simulink library "forceslib"  (R2019b)
settings: Solver=VariableStepAuto  StartTime=0.0  StopTime=10.0  RelTol=1e-3
undefined symbols (not defined in the file or in its folder): MV0, X0
settings Model: Creator=rchen  LastModifiedBy=j-hho

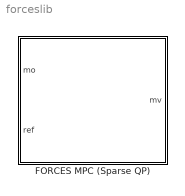
== system forceslib ==
  FORCES MPC (Sparse QP) : Subsystem  InitFcn=forcesmpcblock_InitFcn  mask(ForcesMPC_SparseQP){CoreData=[], StateData=[], md_inport=off, mv_inport=off, uref_inport=off, state_inport=off, ymin_inport=off, ymax_inport=off, umin_inport=off, umax_inport=off, dumin_inport=off, dumax_inport=off, ywt_inport=off, uwt_inport=off, duwt_inport=off, ecrwt_inport=off, return_cost=off, return_mvseq=off, return_qpstatus=off, return_xseq=off, return_state=off, return_yseq=off}
      mask prompts: CoreData "Core Data"; StateData "Initial State Data"; md_inport "Measured disturbance (md)"; mv_inport "External manipulated variable (ext.mv)"; uref_inport "References for manipulated variables (mv.target)"; state_inport "Use custom state estimation (x[k|k])"; ymin_inport "Lower OV Limits (ymin)"; ymax_inport "Upper OV Limits (ymax)"; umin_inport "Lower MV Limits (umin)"; umax_inport "Upper MV Limits (umax)"; dumin_inport "Lower MVRate Limits (dumin)"; dumax_inport "Upper MVRate Limits (dumax)"; ywt_inport "OV Weights (y.wt)"; uwt_inport "MV Weights (u.wt)"; duwt_inport "MVRate Weights (du.wt)"; ecrwt_inport "Slack Variable Weight (ecr.wt)"; return_cost "Optimal cost (cost)"; return_mvseq "Optimal control sequence (mv.seq)"; return_qpstatus "Optimization status (qp.status)"; return_xseq "Optimal state sequence (x.seq)"; return_state "Estimated current states (est.state)"; return_yseq "Optimal output sequence (y.seq)"
      mask help:
      | Simulate MPC controller and generate code  using FORCES QP solver.
      |
      | In MATLAB, use the following commands to generate custom FORCES QP solver from your MPC controller (mpcobj):
      |     options = mpcToForcesOptions('sparse');
      |     [coredata, statedata, onlinedata] = mpcToForces(mpcobj, options);
      | You can enable additional online features via the "options".
      |
      | Afterwards, specify "coredata" and "statedata" in the block dialog and enable additional input and output signals in the block that must be consistent with "options".
      mask init:
      | [blk, Ts, MPCstruct, X0, MV0] = forcesmpcblock_MaskInitFcnParameter;
      | if isempty(MPCstruct)
      |     forcesmpcblock_MaskInitFcnResize(blk,0,1,1,1);
      | else
      |     forcesmpcblock_MaskInitFcnResize(blk,MPCstruct.nmd,MPCstruct.nmv,MPCstruct.ny,MPCstruct.nmy);
      | end
      mask DialogControl Container5 Prompt: Additional Signal Configuration
      mask DialogControl Container7 Prompt: State Estimation
      mask DialogControl Container3 Prompt: Online Constraints
      mask DialogControl Container4 Prompt: Online Weights
      mask DialogControl Container9 Prompt: Additional Output Signals
      mask Display:
      | fprintf('FORCES MPC\n\n(Sparse QP)');
      | port_label('output', 1, 'mv')
      | port_label('input', 1, 'mo')
      | port_label('input', 2, 'ref')

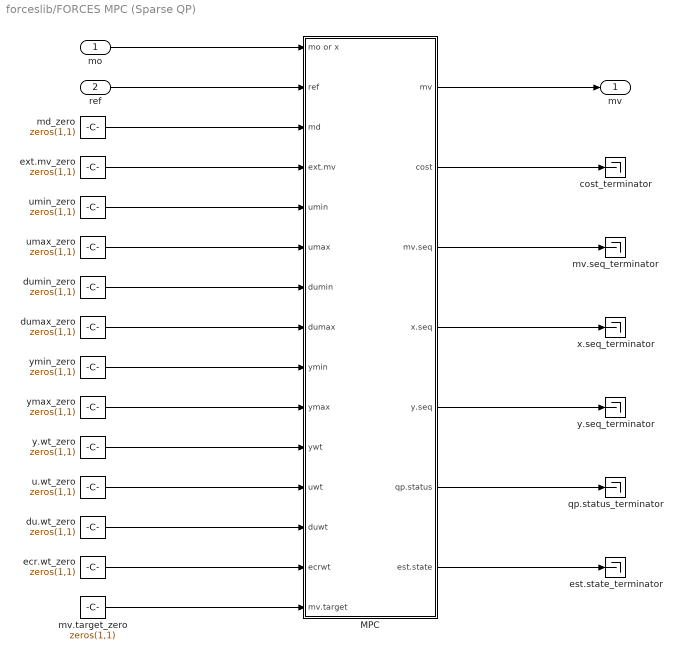
== system forceslib/FORCES MPC (Sparse QP) ==
  mo : Inport
  ref : Inport  Port=2
  MPC : Subsystem
  cost_terminator : Terminator
  du.wt_zero : Constant  Value=zeros(1,1)  SampleTime=-1
  dumax_zero : Constant  Value=zeros(1,1)  SampleTime=-1
  dumin_zero : Constant  Value=zeros(1,1)  SampleTime=-1
  ecr.wt_zero : Constant  Value=zeros(1,1)  SampleTime=-1
  est.state_terminator : Terminator
  ext.mv_zero : Constant  Value=zeros(1,1)  SampleTime=-1
  md_zero : Constant  Value=zeros(1,1)  SampleTime=-1
  mv.seq_terminator : Terminator
  mv.target_zero : Constant  Value=zeros(1,1)  SampleTime=-1
  qp.status_terminator : Terminator
  u.wt_zero : Constant  Value=zeros(1,1)  SampleTime=-1
  umax_zero : Constant  Value=zeros(1,1)  SampleTime=-1
  umin_zero : Constant  Value=zeros(1,1)  SampleTime=-1
  x.seq_terminator : Terminator
  y.seq_terminator : Terminator
  y.wt_zero : Constant  Value=zeros(1,1)  SampleTime=-1
  ymax_zero : Constant  Value=zeros(1,1)  SampleTime=-1
  ymin_zero : Constant  Value=zeros(1,1)  SampleTime=-1
  mv : Outport
  wires:
  mo/1 -> MPC/1(mo or x)
  ref/1 -> MPC/2(ref)
  MPC/1(mv) -> mv/1
  md_zero/1 -> MPC/3(md)
  ext.mv_zero/1 -> MPC/4(ext.mv)
  umin_zero/1 -> MPC/5(umin)
  umax_zero/1 -> MPC/6(umax)
  dumin_zero/1 -> MPC/7(dumin)
  dumax_zero/1 -> MPC/8(dumax)
  ymin_zero/1 -> MPC/9(ymin)
  ymax_zero/1 -> MPC/10(ymax)
  y.wt_zero/1 -> MPC/11(ywt)
  u.wt_zero/1 -> MPC/12(uwt)
  du.wt_zero/1 -> MPC/13(duwt)
  ecr.wt_zero/1 -> MPC/14(ecrwt)
  mv.target_zero/1 -> MPC/15(mv.target)
  MPC/2(cost) -> cost_terminator/1
  MPC/3(mv.seq) -> mv.seq_terminator/1
  MPC/4(x.seq) -> x.seq_terminator/1
  MPC/5(y.seq) -> y.seq_terminator/1
  MPC/6(qp.status) -> qp.status_terminator/1
  MPC/7(est.state) -> est.state_terminator/1

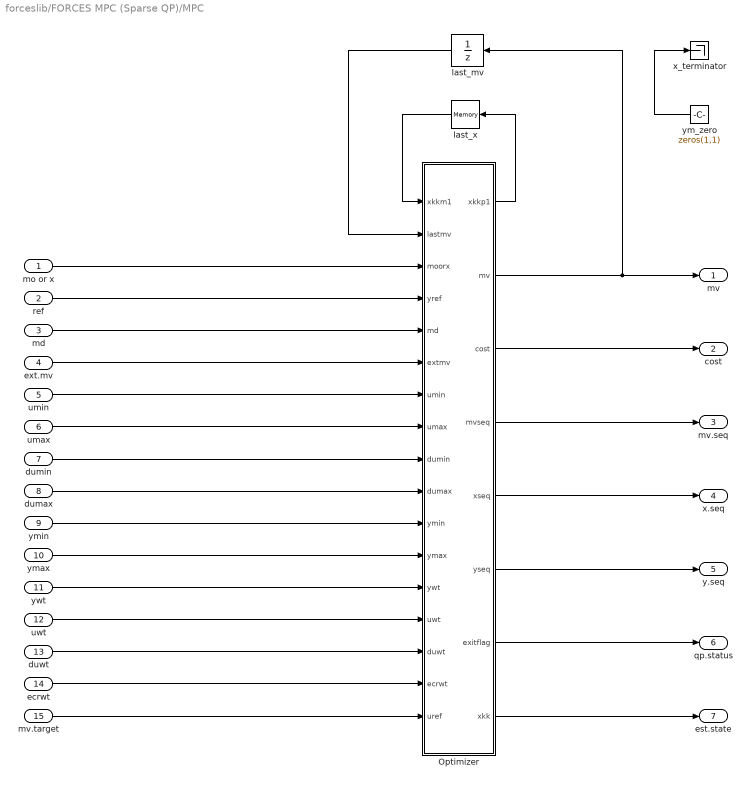
== system forceslib/FORCES MPC (Sparse QP)/MPC ==
  mo or x : Inport
  ref : Inport  Port=2
  md : Inport  Port=3
  ext.mv : Inport  Port=4
  umin : Inport  Port=5
  umax : Inport  Port=6
  dumin : Inport  Port=7
  dumax : Inport  Port=8
  ymin : Inport  Port=9
  ymax : Inport  Port=10
  ywt : Inport  Port=11
  uwt : Inport  Port=12
  duwt : Inport  Port=13
  ecrwt : Inport  Port=14
  mv.target : Inport  Port=15
  Optimizer : MATLAB Function  TreatAsAtomicUnit=on
  last_mv : UnitDelay  InitialCondition=MV0  SampleTime=-1  HasFrameUpgradeWarning=on
  last_x : Memory  InitialCondition=X0  InheritSampleTime=on  LinearizeAsDelay=on
  x_terminator : Terminator
  ym_zero : Constant  Value=zeros(1,1)
  mv : Outport
  cost : Outport  Port=2
  mv.seq : Outport  Port=3
  x.seq : Outport  Port=4
  y.seq : Outport  Port=5
  qp.status : Outport  Port=6
  est.state : Outport  Port=7
  wires:
  mo or x/1 -> Optimizer/3(moorx)
  Optimizer/2(mv) -> last_mv/1, mv/1
  last_x/1 -> Optimizer/1(xkkm1)
  Optimizer/1(xkkp1) -> last_x/1
  last_mv/1 -> Optimizer/2(lastmv)
  ym_zero/1 -> x_terminator/1
  mv.target/1 -> Optimizer/17(uref)
  ecrwt/1 -> Optimizer/16(ecrwt)
  ywt/1 -> Optimizer/13(ywt)
  uwt/1 -> Optimizer/14(uwt)
  duwt/1 -> Optimizer/15(duwt)
  md/1 -> Optimizer/5(md)
  ext.mv/1 -> Optimizer/6(extmv)
  umin/1 -> Optimizer/7(umin)
  umax/1 -> Optimizer/8(umax)
  dumin/1 -> Optimizer/9(dumin)
  dumax/1 -> Optimizer/10(dumax)
  ymin/1 -> Optimizer/11(ymin)
  ymax/1 -> Optimizer/12(ymax)
  Optimizer/8(xkk) -> est.state/1
  Optimizer/7(exitflag) -> qp.status/1
  Optimizer/6(yseq) -> y.seq/1
  Optimizer/5(xseq) -> x.seq/1
  Optimizer/4(mvseq) -> mv.seq/1
  Optimizer/3(cost) -> cost/1
  ref/1 -> Optimizer/4(yref)

== matlab function forceslib/FORCES MPC (Sparse QP)/MPC/Optimizer ==
  settings: updateMethod=DISCRETE  sampleTime=Ts
  data: xkkm1 input double; lastmv input; xkkp1 output; moorx input; mv output; yref input; md input; extmv input; umin input; umax input; dumin input; dumax input; ymin input; ymax input; ywt input; uwt input; duwt input; ecrwt input; uref input; MPCstruct parameter; cost output; mvseq output; xseq output; yseq output; exitflag output; xkk output
function [xkkp1,mv,cost,mvseq,xseq,yseq,exitflag,xkk] = fcn(xkkm1,lastmv,moorx,yref,md,extmv,umin,umax,dumin,dumax,ymin,ymax,ywt,uwt,duwt,ecrwt,uref,MPCstruct)
% Pre-allocate all the MEX block outputs for the simulation mode %#ok<*PREALL>
if isempty(MPCstruct)
    [xkkp1,mv,cost,mvseq,xseq,yseq,exitflag,xkk]= deal(0);
else
    %% states
    statedata.Plant = reshape(xkkm1(1:MPCstruct.nxp),MPCstruct.nxp,1);
    statedata.Disturbance = reshape(xkkm1(MPCstruct.nxp+1:MPCstruct.nxp+MPCstruct.nxdist),MPCstruct.nxdist,1);
    statedata.Noise = reshape(xkkm1(MPCstruct.nxp+MPCstruct.nxdist+1:MPCstruct.nxp+MPCstruct.nxdist+MPCstruct.nxnoise),MPCstruct.nxnoise,1);
    statedata.LastMove = reshape(lastmv,MPCstruct.nmv,1);
    %% ref
    onlinedata.signals.ref = reshape(yref,numel(yref)/MPCstruct.ny,MPCstruct.ny);
    %% md if requested
    if MPCstruct.nmd>0
        onlinedata.signals.md = reshape(md,numel(md)/MPCstruct.nmd,MPCstruct.nmd);
    end
    %% ym if built-in estimation is used
    if ~MPCstruct.IsCustomEstimation
        onlinedata.signals.ym = reshape(moorx,MPCstruct.nmy,1);
    end
    %% externalMV if requested
    if MPCstruct.UseExternalMV
        onlinedata.signals.externalMV = reshape(extmv,MPCstruct.nmv,1);
    end
    %% mvTarget if requested
    if MPCstruct.UseMVTarget
        onlinedata.signals.mvTarget = reshape(uref,numel(uref)/MPCstruct.nmv,MPCstruct.nmv);
    end
    %% weights
    if MPCstruct.UseOnlineWeightOV
        onlinedata.weights.y = appendRows(ywt,MPCstruct.p,MPCstruct.ny);
    end
    if MPCstruct.UseOnlineWeightMV
        onlinedata.weights.u = appendRows(uwt,MPCstruct.p,MPCstruct.nmv);
    end
    if MPCstruct.UseOnlineWeightMVRate
        onlinedata.weights.du = appendRows(duwt,MPCstruct.p,MPCstruct.nmv);
    end
    if MPCstruct.UseOnlineWeightECR
        onlinedata.weights.ecr = ecrwt;
    end
    %% constraints
    if MPCstruct.UseOnlineConstraintOVMax
        onlinedata.limits.ymax = appendRows(ymax,MPCstruct.p,MPCstruct.ny);
    end
    if MPCstruct.UseOnlineConstraintOVMin
        onlinedata.limits.ymin = appendRows(ymin,MPCstruct.p,MPCstruct.ny);
    end
    if MPCstruct.UseOnlineConstraintMVMax
        onlinedata.limits.umax = appendRows(umax,MPCstruct.p,MPCstruct.nmv);
    end
    if MPCstruct.UseOnlineConstraintMVMin
        onlinedata.limits.umin = appendRows(umin,MPCstruct.p,MPCstruct.nmv);
    end
    if MPCstruct.UseOnlineConstraintMVRateMax
        onlinedata.limits.dumax = appendRows(dumax,MPCstruct.p,MPCstruct.nmv);
    end
    if MPCstruct.UseOnlineConstraintMVRateMin
        onlinedata.limits.dumin = appendRows(dumin,MPCstruct.p,MPCstruct.nmv);
    end
    mv = lastmv;
    newstatedata = statedata;
    info = struct('Uopt',zeros(MPCstruct.p,MPCstruct.nmv),...
                  'DUopt',zeros(MPCstruct.p,MPCstruct.nmv),...
                  'Yopt',zeros(MPCstruct.p,MPCstruct.ny),...
                  'Xopt',zeros(MPCstruct.p,MPCstruct.nxQP),...
                  'Slack',zeros(MPCstruct.p,1),...
                  'ExitFlag',0,...
                  'Iterations',0,...
                  'Cost',0);
    [mv, newstatedata, info] = mpcmoveForces(MPCstruct, statedata, onlinedata);
    xkkp1 = [newstatedata.Plant;newstatedata.Disturbance;newstatedata.Noise];
    cost = info.Cost;
    mvseq = info.Uopt;
    xseq = info.Xopt;
    yseq = info.Yopt;
    exitflag = info.ExitFlag;
    xkk = info.CurrentState;
end

function val = appendRows(data,p,cols)
rows0 = numel(data)/cols;
val0 = reshape(data,rows0,cols);
val = zeros(p,cols);
for ct=1:p
    val(ct,:) = val0(min(rows0,ct),:);
end
